simulink model "Sq_wave"  (R2019a)
settings: Solver=ode45  StartTime=0.0  StopTime=0.2  MaxStep=1e-4  RelTol=1e-3
values from neighbouring files (symbols this model uses):
  f = 50    [inputs.m]
  L = 33e-3    (= 0.033)    [inputs.m]
  R = 33    [inputs.m]
  Vdc = 100    [inputs.m]
libraries: powerlib x10
settings Model: Creator=omar_  LastModifiedBy=omar_
settings DataIOCC: ReturnWorkspaceOutputs=off

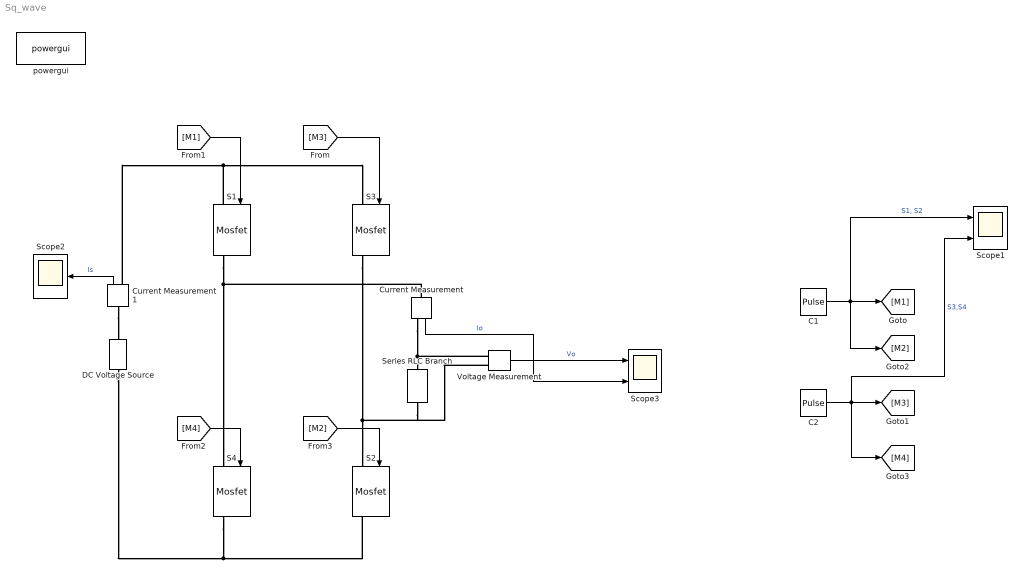
== system Sq_wave ==
  C1 : DiscretePulseGenerator  PulseType=Time based  Period=1/f  PulseWidth=50
  C2 : DiscretePulseGenerator  PulseType=Time based  Period=1/f  PulseWidth=50  PhaseDelay=1/(2*f)
  Current Measurement : powerlib/Measurements/Current Measurement  PhasorSimulation=off  OutputType=Magnitude  PSBequivalent=0
      settings: SourceProductName=Simscape Electrical
  Current Measurement1 : powerlib/Measurements/Current Measurement  PhasorSimulation=off  OutputType=Magnitude  PSBequivalent=0
      settings: SourceProductName=Simscape Electrical
  DC Voltage Source : powerlib/Electrical Sources/DC Voltage Source  Amplitude=Vdc  Measurements=None
      settings: SourceProductName=Simscape Electrical
  S{1..4} (4 alike) : powerlib/Power Electronics/Mosfet  Ron=0.1  Lon=0  Rd=0.01  Vfd=0  IC=0  Rs=1e5  Cs=inf  Measurements=on
      settings: SourceProductName=Simscape Electrical
  Scope1 : Scope  NumInputPorts=2
  Scope2 : Scope
  Scope3 : Scope  NumInputPorts=2
  Series RLC Branch : powerlib/Elements/Series RLC Branch  LConnTagsString=__new0  RConnTagsString=__new0  BranchType=RL  Resistance=R  Inductance=L  SetiL0=off  InitialCurrent=0  Capacitance=1e-6  Setx0=off  InitialVoltage=0  Measurements=None
      settings: SourceProductName=Simscape Electrical
  Voltage Measurement : powerlib/Measurements/Voltage Measurement  PhasorSimulation=off  OutputType=Magnitude  PSBequivalent=0
      settings: SourceProductName=Simscape Electrical
  powergui : powerlib/powergui  Priority=1  SimulationMode=Continuous  SampleTime=1e-6  frequency=60  Iterations=50  frequencyindice=0  Pbase=100e6  ErrMax=1e-4  UnitsV=kV  UnitsW=MW  buscounter=0  FunctionMessages=off  echomessages=off  EnableUseOfTLC=off  CurrentSourceSwitches=off  DisableSnubberDevices=off  DisableRonSwitches=off  DisableVfSwitches=off  DisplayEquations=off  AutomaticDiscreteSolvers=off  SolverType=Tustin/Backward Euler (TBE)  Interpol=off  ExternalGateDelay=off  methode=off  Ts=100  x0status=blocks  SPID=on  SwTol=0  HookPort=off  NonlinearTolerance=0  nMaxIteration=15  ContinueOnMaxIteration=off  RestoreLinks=warning  ResistiveCurrentMeasurement=off  Frange=[0:2:500]  Ylog=off  Xlog=on  ShowGrid=off  save=off  variable=ZData  structure=Outputs  ZoomFFT=off  StartTime=0.08  cycles=3  DisplayStyle=2  fundamental=50  FreqAxis=off  MaxFrequency=1000  frequencyindicesteady=1  RmsSteady=1  display=off
      settings: SourceProductName=Simscape Electrical
  wires:
  Voltage Measurement/1 -> Scope3/1  "Vo"
  Current Measurement1/1 -> Scope2/1  "Is"
  Current Measurement/1 -> Scope3/2  "Io"
  [M1] -> S1/1
  [M3] -> S3/1
  [M4] -> S4/1
  [M2] -> S2/1
  C2/1 -> Scope1/2, [M4], [M3]  "S3,S4"
  C1/1 -> [M2], Scope1/1, [M1]  "S1, S2"
  connections:
  Current Measurement1/RConn1 -- S1/LConn1 -- S3/LConn1
  S1/RConn1 -- S4/LConn1 -- Current Measurement/LConn1
  S4/RConn1 -- DC Voltage Source/LConn1 -- S2/RConn1
  S3/RConn1 -- Series RLC Branch/RConn1 -- Voltage Measurement/LConn2 -- S2/LConn1
  Current Measurement/RConn1 -- Voltage Measurement/LConn1 -- Series RLC Branch/LConn1
  Current Measurement1/LConn1 -- DC Voltage Source/RConn1
